simulink subsystem "SimulinkPlantModels"  (R2022b)
settings: Solver=VariableStepAuto  StartTime=0.0  StopTime=10.0  RelTol=1e-3
undefined symbols (not defined in the file): PlntDCDCVoltInit, PlntTrnsfrCaseAxlSpdLock, PlntTrnsfrCaseTrqSplitRatio
libraries: vehdynlibsens x1
(part 2 of 2)

== system SimulinkPlantModels/Electrical System/Electrical System 1EM/Electric Machine 1 ==
  EMTrqCmd : Inport
  EMSpd : Inport  Port=2
  BusVolt : Inport  Port=3
  Mapped EM : Subsystem  VariantControl=Mapped EM  ReferencedSubsystem=ElectricMachine1
  EMTrq : Outport  VectorParamsAs1DForOutWhenUnconnected=off
  EMCurr : Outport  Port=2  VectorParamsAs1DForOutWhenUnconnected=off

== system SimulinkPlantModels/Electrical System/Electrical System 2EM/Battery System ==
  note: 1) Add Subsystem or Model blocks as valid variant choices.
      | 2) You cannot connect blocks at this level. At simulation, connectivity is automatically
      | determined, based on the active variant and port name matching.
  LdCurr : Inport
  BattTemp : Inport  Port=2
  Ideal Voltage Source : Subsystem  VariantControl=Ideal Voltage Source  ReferencedSubsystem=IdealVoltageSource
  Mapped Battery : Subsystem  VariantControl=Mapped Battery  ReferencedSubsystem=Battery
  BattSoc : Outport  VectorParamsAs1DForOutWhenUnconnected=off
  BattCurr : Outport  Port=2  VectorParamsAs1DForOutWhenUnconnected=off
  BattVolt : Outport  Port=3  VectorParamsAs1DForOutWhenUnconnected=off
  BMSSensors : Outport  Port=4  VectorParamsAs1DForOutWhenUnconnected=off

== system SimulinkPlantModels/Electrical System/Electrical System 2EM/DC-DC Converter ==
  BatVolt : Inport
  LdCurr : Inport  Port=2
  VoltCmd : Inport  Port=3
  DC-DC Converter : Subsystem  VariantControl=DC-DC Converter  ReferencedSubsystem=DCDCConverter
  No DC-DC Converter : Subsystem  VariantControl=No DC-DC Converter  ReferencedSubsystem=NoDCDCConverter
  BusVolt : Outport
  SrcCurr : Outport  Port=2

== system SimulinkPlantModels/Electrical System/Electrical System 2EM/Electric Machine 1 ==
  EMTrqCmd : Inport
  EMSpd : Inport  Port=2
  BusVolt : Inport  Port=3
  Mapped EM : Subsystem  VariantControl=Mapped EM  ReferencedSubsystem=ElectricMachine1
  EMTrq : Outport  VectorParamsAs1DForOutWhenUnconnected=off
  EMCurr : Outport  Port=2  VectorParamsAs1DForOutWhenUnconnected=off

== system SimulinkPlantModels/Electrical System/Electrical System 2EM/Electric Machine 2 ==
  EMTrqCmd : Inport
  EMSpd : Inport  Port=2
  BusVolt : Inport  Port=3
  Mapped EM : Subsystem  VariantControl=Mapped EM  ReferencedSubsystem=ElectricMachine2
  EMTrq : Outport  VectorParamsAs1DForOutWhenUnconnected=off
  EMCurr : Outport  Port=2  VectorParamsAs1DForOutWhenUnconnected=off

== system SimulinkPlantModels/Sensors/Sensors/IMU Sensor ==
  VehFdbk : Inport
  Bus Creator1 : BusCreator  Inputs=2
  Bus Selector : BusSelector  OutputSignals=BdyFrm.Cg.Acc.ax,BdyFrm.Cg.Acc.ay,BdyFrm.Cg.Acc.az  OutputAsBus=on
  Bus Selector1 : BusSelector  OutputSignals=BdyFrm.Cg.AngVel.p,BdyFrm.Cg.AngVel.q,BdyFrm.Cg.AngVel.r  OutputAsBus=on
  Bus Selector2 : BusSelector  OutputSignals=BdyFrm.Cg.AngAcc.pdot,BdyFrm.Cg.AngAcc.qdot,BdyFrm.Cg.AngAcc.rdot  OutputAsBus=on
  Bus to Vector : BusToVector
  Bus to Vector1 : BusToVector
  Bus to Vector2 : BusToVector
  Constant : Constant  Value=[0,0,0]  SampleTime=-1
  Constant1 : Constant  Value=[0,0,9.81]  SampleTime=-1
  Three-axis Inertial Measurement Unit : vehdynlibsens/Three-axis Inertial Measurement Unit  units=Metric (MKS)  imu=[0 0 0]  i_Ts=0  dtype_a=off  w_a=190  z_a=0.707  a_sf_cc=[1 0 0; 0 1 0; 0 0 1]  a_bias=[0 0 0]  a_sat="[-inf  -inf  -inf  inf inf inf]"  dtype_g=off  w_g=190  z_g=0.707  g_sf_cc=[1 0 0; 0 1 0; 0 0 1]  g_bias=[0 0 0]  g_sens=[0 0 0]  g_sat="[-inf  -inf  -inf  inf inf inf]"  i_rand=on  i_seeds=[23093 23094 23095 23096 23097 23098]  i_pow=[0.001 0.001 0.001 0.0001 0.0001 0.0001]  aMode=2
  Unit Conversion : UnitConversion
  IMU : Outport
  wires:
  VehFdbk/1 -> Bus Selector/1, Bus Selector1/1, Bus Selector2/1
  Constant1/1 -> Three-axis Inertial Measurement Unit/5
  Bus to Vector/1 -> Unit Conversion/1
  Bus Selector1/1 -> Bus to Vector1/1
  Bus to Vector1/1 -> Three-axis Inertial Measurement Unit/2
  Bus Selector/1 -> Bus to Vector/1
  Bus to Vector2/1 -> Three-axis Inertial Measurement Unit/3
  Three-axis Inertial Measurement Unit/1 -> Bus Creator1/1  "Acc"
  Bus Creator1/1 -> IMU/1  "IMU"
  Bus Selector2/1 -> Bus to Vector2/1
  Constant/1 -> Three-axis Inertial Measurement Unit/4
  Three-axis Inertial Measurement Unit/2 -> Bus Creator1/2  "pqr"
  Unit Conversion/1 -> Three-axis Inertial Measurement Unit/1

== system SimulinkPlantModels/Sensors/Sensors/No IMU Sensor ==
  VehFdbk : Inport
  Bus Creator1 : BusCreator  Inputs=2
  Constant : Constant  Value=zeros(3,1)  SampleTime=-1
  Constant1 : Constant  Value=zeros(3,1)  SampleTime=-1
  Terminator : Terminator
  IMU : Outport
  wires:
  VehFdbk/1 -> Terminator/1
  Constant1/1 -> Bus Creator1/2  "pqr"
  Bus Creator1/1 -> IMU/1  "IMU"
  Constant/1 -> Bus Creator1/1  "Acc"

== system SimulinkPlantModels/Drivetrain/Transmission and Actuators/Conventional Vehicle/Transmission ==
  GearCmd : Inport
  EngTrq : Inport  Port=2
  DriveshftSpd : Inport  Port=3
  Automated Manual Transmission : Subsystem  VariantControl=Automated Manual Transmission  ReferencedSubsystem=AutomatedManualTransmission
  Automatic Transmission With Torque Converter : Subsystem  VariantControl=Automatic Transmission With Torque Converter  ReferencedSubsystem=AutomaticTransmissionWithTorqueConverter
  Ideal Fixed Gear Transmission : Subsystem  VariantControl=Ideal Fixed Gear Transmission  ReferencedSubsystem=IdealFixedGearTransmission
  Cltch2State : Outport
  Info : Outport  Port=2
  EngSpd : Outport  Port=3
  DriveshftTrq : Outport  Port=4
